simulink model "KalmanFilter(1)"  (R2024a)
settings: Solver=VariableStepAuto  StartTime=0.0  StopTime=1  RelTol=1e-3

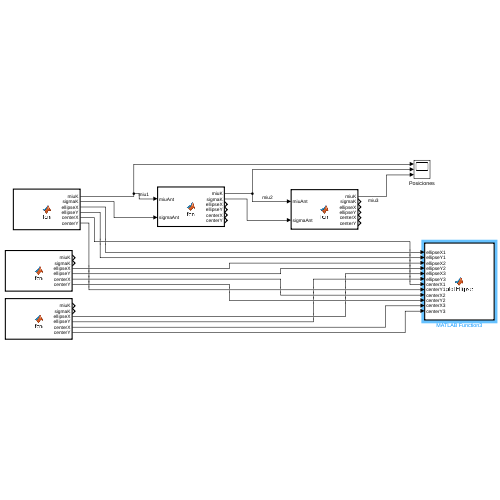
[thumbnail: Simulink's stored preview of the top-level diagram]
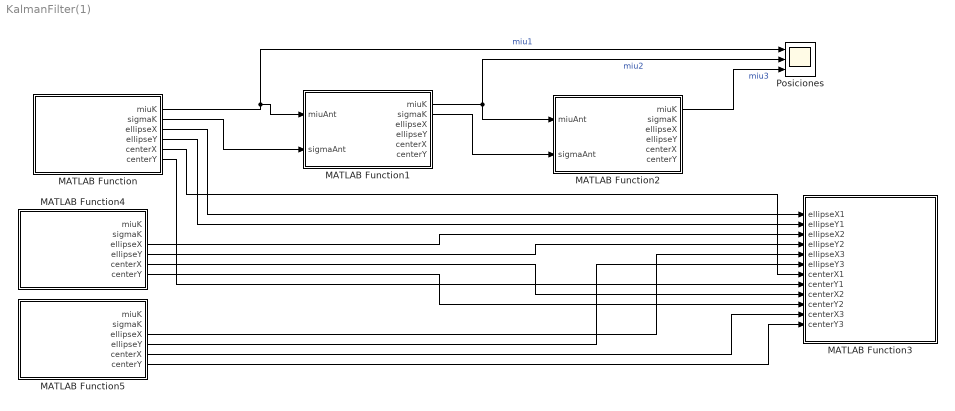
== system KalmanFilter(1) ==
  MATLAB Function : MATLAB Function  TreatAsAtomicUnit=on
  MATLAB Function1 : MATLAB Function  TreatAsAtomicUnit=on
  MATLAB Function2 : MATLAB Function  TreatAsAtomicUnit=on
  MATLAB Function3 : MATLAB Function  TreatAsAtomicUnit=on
  MATLAB Function4 : MATLAB Function  TreatAsAtomicUnit=on
  MATLAB Function5 : MATLAB Function  TreatAsAtomicUnit=on
  Posiciones : Scope  NumInputPorts=3
  wires:
  MATLAB Function/1(miuK) -> Posiciones/1, MATLAB Function1/1(miuAnt)  "miu1"
  MATLAB Function/2(sigmaK) -> MATLAB Function1/2(sigmaAnt)
  MATLAB Function1/1(miuK) -> Posiciones/2, MATLAB Function2/1(miuAnt)  "miu2"
  MATLAB Function1/2(sigmaK) -> MATLAB Function2/2(sigmaAnt)
  MATLAB Function2/1(miuK) -> Posiciones/3  "miu3"
  MATLAB Function/3(ellipseX) -> MATLAB Function3/1(ellipseX1)
  MATLAB Function/4(ellipseY) -> MATLAB Function3/2(ellipseY1)
  MATLAB Function/5(centerX) -> MATLAB Function3/7(centerX1)
  MATLAB Function/6(centerY) -> MATLAB Function3/8(centerY1)
  MATLAB Function4/3(ellipseX) -> MATLAB Function3/3(ellipseX2)
  MATLAB Function4/4(ellipseY) -> MATLAB Function3/4(ellipseY2)
  MATLAB Function4/5(centerX) -> MATLAB Function3/9(centerX2)
  MATLAB Function4/6(centerY) -> MATLAB Function3/10(centerY2)
  MATLAB Function5/3(ellipseX) -> MATLAB Function3/5(ellipseX3)
  MATLAB Function5/4(ellipseY) -> MATLAB Function3/6(ellipseY3)
  MATLAB Function5/5(centerX) -> MATLAB Function3/11(centerX3)
  MATLAB Function5/6(centerY) -> MATLAB Function3/12(centerY3)

== matlab function KalmanFilter(1)/MATLAB Function1 ==
  data: miuK output; sigmaK output; miuAnt input; sigmaAnt input; ellipseX output; ellipseY output; centerX output; centerY output
function [miuK, sigmaK, ellipseX, ellipseY, centerX, centerY]= fcn (miuAnt, sigmaAnt)

m = [3; 4]                      %Landmark position

QK = [0.5  0.01 0.01;           %Covariance Matrix - Motion(encoders)
      0.01 0.5  0.01;
      0.01 0.01 0.2]

RK = [0.1 0;                    %Covariance Matrix - Observation(LiDAR)
      0   0.02]
VK = 4 % m/s
WK = 4 % rad/s
deltaT = 0.1      %Time Sampling

z12 = [4.72; 0.72]
z13 = [4.69; 0.65]

%Step 2
miuK_est = [miuAnt(1) + deltaT * VK * cos(miuAnt(3));
            miuAnt(2) + deltaT * VK * sin(miuAnt(3));
            miuAnt(3) + deltaT * WK]
%Step 3
HK = [1 0 -deltaT * VK *sin(miuAnt(3));
      0 1 deltaT * VK *cos(miuAnt(3));
      0 0 1]

%Step 4 - Propagation of uncertainty
SigmaK = HK * sigmaAnt * HK' + QK

%Step 6 - Position Difference / Observation Model
deltaX = m(1) - miuK_est(1)
deltaY = m(2) - miuK_est(2)
p = (deltaX * deltaX) + (deltaY * deltaY)

ZK_est = [sqrt(p);                              
          atan2(deltaY, deltaX) - miuK_est(3)] 

%Step 7 - Linearise the observation model
GK = [-deltaX/sqrt(p) -deltaY/sqrt(p) 0;
      deltaY/p        -deltaX/p      -1]

%Step 8 - Second uncertainty Propagation
ZK = GK * SigmaK * GK' + RK

%Step 9 - Kalman Gain
Kk = SigmaK * GK' * inv(ZK)

%Step 10 - Position Calculation using real observation
miuK = miuK_est + Kk * (z12 -ZK_est)

%Step 11 - Get covariance
sigmaK = (eye(3) - Kk * GK) * QK

[ellipseX, ellipseY] = calculateEllipse(miuK(1:2), sigmaK(1:2, 1:2));
centerX = miuK(1);
centerY = miuK(2);
end

function [ellipseX, ellipseY] = calculateEllipse(mu, Sigma)
    theta = linspace(0, 2*pi, 100);
    [eig_vec, eig_val] = eig(Sigma);
    ellipse_points = [cos(theta); sin(theta)]' * sqrt(eig_val) * eig_vec';
    ellipseX = ellipse_points(:,1) + mu(1);
    ellipseY = ellipse_points(:,2) + mu(2);
end

== matlab function KalmanFilter(1)/MATLAB Function ==
  data: miuK output; sigmaK output; ellipseX output; ellipseY output; centerX output; centerY output
function [miuK, sigmaK, ellipseX, ellipseY, centerX, centerY]= fcn

%Miu = Position
miuAnt = [0; 0; 0]              %Robot First position
sigmaAnt = [0 0 0 ;             %Initial covariance matrix
            0 0 0; 
            0 0 0]              
m = [3; 4]                      %Landmark position

QK = [0.5  0.01 0.01;           %Covariance Matrix - Motion(encoders)
      0.01 0.5  0.01;
      0.01 0.01 0.2]

RK = [0.1 0;                    %Covariance Matrix - Observation(LiDAR)
      0   0.02]
VK = 1 % m/s
WK = 1 % rad/s
deltaT = 0.1      %Time Sampling

z11 = [4.87; 0.8]
z12 = [4.72; 0.72]
z13 = [4.69; 0.65]

%Step 2
miuK_est = [miuAnt(1) + deltaT * VK * cos(miuAnt(3));
            miuAnt(2) + deltaT * VK * sin(miuAnt(3));
            miuAnt(3) + deltaT * WK]
%Step 3
HK = [1 0 -deltaT * VK *sin(miuAnt(3));
      0 1 deltaT * VK *cos(miuAnt(3));
      0 0 1]

%Step 4 - Propagation of uncertainty
SigmaK = HK * sigmaAnt * HK' + QK

%Step 6 - Position Difference / Observation Model
deltaX = m(1) - miuK_est(1)
deltaY = m(2) - miuK_est(2)
p = (deltaX * deltaX) + (deltaY * deltaY)

ZK_est = [sqrt(p);                              
          atan2(deltaY, deltaX) - miuK_est(3)] 

%Step 7 - Linearise the observation model
GK = [-deltaX/sqrt(p) -deltaY/sqrt(p) 0;
      deltaY/p        -deltaX/p      -1]

%Step 8 - Second uncertainty Propagation
ZK = GK * SigmaK * GK' + RK

%Step 9 - Kalman Gain
Kk = SigmaK * GK' * inv(ZK)
%Step 10 - Position Calculation using real observation
miuK = miuK_est + Kk * (z11 -ZK_est)

%Step 11 - Get covariance
sigmaK = (eye(3) - Kk * GK) * QK

[ellipseX, ellipseY] = calculateEllipse(miuK(1:2), sigmaK(1:2, 1:2));
centerX = miuK(1);
centerY = miuK(2);
end

function [ellipseX, ellipseY] = calculateEllipse(mu, Sigma)
    theta = linspace(0, 2*pi, 100);
    [eig_vec, eig_val] = eig(Sigma);
    ellipse_points = [cos(theta); sin(theta)]' * sqrt(eig_val) * eig_vec';
    ellipseX = ellipse_points(:,1) + mu(1);
    ellipseY = ellipse_points(:,2) + mu(2);
end

== matlab function KalmanFilter(1)/MATLAB Function2 ==
  data: miuK output; sigmaK output; miuAnt input; sigmaAnt input; ellipseX output; ellipseY output; centerX output; centerY output
function [miuK, sigmaK, ellipseX, ellipseY, centerX, centerY]= fcn (miuAnt, sigmaAnt)

m = [3; 4]                      %Landmark position

QK = [0.5  0.01 0.01;           %Covariance Matrix - Motion(encoders)
      0.01 0.5  0.01;
      0.01 0.01 0.2]

RK = [0.1 0;                    %Covariance Matrix - Observation(LiDAR)
      0   0.02]
VK = 4 % m/s
WK = 4 % rad/s
deltaT = 0.1      %Time Sampling

z13 = [4.69; 0.65]

%Step 2
miuK_est = [miuAnt(1) + deltaT * VK * cos(miuAnt(3));
            miuAnt(2) + deltaT * VK * sin(miuAnt(3));
            miuAnt(3) + deltaT * WK]
%Step 3
HK = [1 0 -deltaT * VK *sin(miuAnt(3));
      0 1 deltaT * VK *cos(miuAnt(3));
      0 0 1]

%Step 4 - Propagation of uncertainty
SigmaK = HK * sigmaAnt * HK' + QK

%Step 6 - Position Difference / Observation Model
deltaX = m(1) - miuK_est(1)
deltaY = m(2) - miuK_est(2)
p = (deltaX * deltaX) + (deltaY * deltaY)

ZK_est = [sqrt(p);                              
          atan2(deltaY, deltaX) - miuK_est(3)] 

%Step 7 - Linearise the observation model
GK = [-deltaX/sqrt(p) -deltaY/sqrt(p) 0;
      deltaY/p        -deltaX/p      -1]

%Step 8 - Second uncertainty Propagation
ZK = GK * SigmaK * GK' + RK

%Step 9 - Kalman Gain
Kk = SigmaK * GK' * inv(ZK)

%Step 10 - Position Calculation using real observation
miuK = miuK_est + Kk * (z13 -ZK_est)

%Step 11 - Get covariance
sigmaK = (eye(3) - Kk * GK) * QK

[ellipseX, ellipseY] = calculateEllipse(miuK(1:2), sigmaK(1:2, 1:2));
centerX = miuK(1);
centerY = miuK(2);
end

function [ellipseX, ellipseY] = calculateEllipse(mu, Sigma)
    theta = linspace(0, 2*pi, 100);
    [eig_vec, eig_val] = eig(Sigma);
    ellipse_points = [cos(theta); sin(theta)]' * sqrt(eig_val) * eig_vec';
    ellipseX = ellipse_points(:,1) + mu(1);
    ellipseY = ellipse_points(:,2) + mu(2);
end

== matlab function KalmanFilter(1)/MATLAB Function3 ==
  data: ellipseX1 input; ellipseY1 input; ellipseX2 input; ellipseY2 input; ellipseX3 input; ellipseY3 input; centerX1 input; centerY1 input; centerX2 input; centerY2 input; centerX3 input; centerY3 input
function plotEllipse(ellipseX1, ellipseY1, ellipseX2, ellipseY2, ellipseX3, ellipseY3, centerX1, centerY1, centerX2, centerY2, centerX3, centerY3)
    % Check if the figure is already open
    existing_figures = findall(0, 'Type', 'figure');
    if isempty(existing_figures)
        figure;
    else
        figure(existing_figures(1)); % Use the first existing figure
    end
    
    hold on;
    
    % Plot the first ellipse
    plot(ellipseX1, ellipseY1, 'b-');
    plot(centerX1, centerY1, 'bo', 'MarkerSize', 10, 'LineWidth', 2); % Centro de la elipse 1
    
    % Plot the second ellipse
    plot(ellipseX2, ellipseY2, 'r-');
    plot(centerX2, centerY2, 'ro', 'MarkerSize', 10, 'LineWidth', 2); % Centro de la elipse 2
    
    % Plot the third ellipse
    plot(ellipseX3, ellipseY3, 'g-');
    plot(centerX3, centerY3, 'go', 'MarkerSize', 10, 'LineWidth', 2); % Centro de la elipse 3
    
    hold off;
    xlabel('X');
    ylabel('Y');
    title('Confidence Ellipses');
    axis equal;
    grid on;
    legend('Ellipse 1 - Original', 'Center 1', 'Ellipse 2 - Qk Double Values', 'Center 2', 'Ellipse 3 - Rk double values', 'Center 3');
end

== matlab function KalmanFilter(1)/MATLAB Function4 ==
  data: miuK output; sigmaK output; ellipseX output; ellipseY output; centerX output; centerY output
function [miuK, sigmaK, ellipseX, ellipseY, centerX, centerY]= fcn

%Miu = Position
miuAnt = [0; 0; 0]              %Robot First position
sigmaAnt = [0 0 0 ;             %Initial covariance matrix
            0 0 0; 
            0 0 0]              
m = [3; 4]                      %Landmark position

QK = [1.0  0.01 0.01;           %Covariance Matrix - Motion(encoders)
      0.01 1.0  0.01;
      0.01 0.01 0.4]

RK = [0.1 0;                    %Covariance Matrix - Observation(LiDAR)
      0   0.02]
VK = 1 % m/s
WK = 1 % rad/s
deltaT = 0.1      %Time Sampling

z11 = [4.87; 0.8]
z12 = [4.72; 0.72]
z13 = [4.69; 0.65]

%Step 2
miuK_est = [miuAnt(1) + deltaT * VK * cos(miuAnt(3));
            miuAnt(2) + deltaT * VK * sin(miuAnt(3));
            miuAnt(3) + deltaT * WK]
%Step 3
HK = [1 0 -deltaT * VK *sin(miuAnt(3));
      0 1 deltaT * VK *cos(miuAnt(3));
      0 0 1]

%Step 4 - Propagation of uncertainty
SigmaK = HK * sigmaAnt * HK' + QK

%Step 6 - Position Difference / Observation Model
deltaX = m(1) - miuK_est(1)
deltaY = m(2) - miuK_est(2)
p = (deltaX * deltaX) + (deltaY * deltaY)

ZK_est = [sqrt(p);                              
          atan2(deltaY, deltaX) - miuK_est(3)] 

%Step 7 - Linearise the observation model
GK = [-deltaX/sqrt(p) -deltaY/sqrt(p) 0;
      deltaY/p        -deltaX/p      -1]

%Step 8 - Second uncertainty Propagation
ZK = GK * SigmaK * GK' + RK

%Step 9 - Kalman Gain
Kk = SigmaK * GK' * inv(ZK)
%Step 10 - Position Calculation using real observation
miuK = miuK_est + Kk * (z11 -ZK_est)

%Step 11 - Get covariance
sigmaK = (eye(3) - Kk * GK) * QK

[ellipseX, ellipseY] = calculateEllipse(miuK(1:2), sigmaK(1:2, 1:2));
centerX = miuK(1);
centerY = miuK(2);
end

function [ellipseX, ellipseY] = calculateEllipse(mu, Sigma)
    theta = linspace(0, 2*pi, 100);
    [eig_vec, eig_val] = eig(Sigma);
    ellipse_points = [cos(theta); sin(theta)]' * sqrt(eig_val) * eig_vec';
    ellipseX = ellipse_points(:,1) + mu(1);
    ellipseY = ellipse_points(:,2) + mu(2);
end

== matlab function KalmanFilter(1)/MATLAB Function5 ==
  data: miuK output; sigmaK output; ellipseX output; ellipseY output; centerX output; centerY output
function [miuK, sigmaK, ellipseX, ellipseY, centerX, centerY]= fcn

%Miu = Position
miuAnt = [0; 0; 0]              %Robot First position
sigmaAnt = [0 0 0 ;             %Initial covariance matrix
            0 0 0; 
            0 0 0]              
m = [3; 4]                      %Landmark position

QK = [0.5  0.01 0.01;           %Covariance Matrix - Motion(encoders)
      0.01 0.5  0.01;
      0.01 0.01 0.2]

RK = [0.2 0;                    %Covariance Matrix - Observation(LiDAR)
      0   0.04]
VK = 1 % m/s
WK = 1 % rad/s
deltaT = 0.1      %Time Sampling

z11 = [4.87; 0.8]
z12 = [4.72; 0.72]
z13 = [4.69; 0.65]

%Step 2
miuK_est = [miuAnt(1) + deltaT * VK * cos(miuAnt(3));
            miuAnt(2) + deltaT * VK * sin(miuAnt(3));
            miuAnt(3) + deltaT * WK]
%Step 3
HK = [1 0 -deltaT * VK *sin(miuAnt(3));
      0 1 deltaT * VK *cos(miuAnt(3));
      0 0 1]

%Step 4 - Propagation of uncertainty
SigmaK = HK * sigmaAnt * HK' + QK

%Step 6 - Position Difference / Observation Model
deltaX = m(1) - miuK_est(1)
deltaY = m(2) - miuK_est(2)
p = (deltaX * deltaX) + (deltaY * deltaY)

ZK_est = [sqrt(p);                              
          atan2(deltaY, deltaX) - miuK_est(3)] 

%Step 7 - Linearise the observation model
GK = [-deltaX/sqrt(p) -deltaY/sqrt(p) 0;
      deltaY/p        -deltaX/p      -1]

%Step 8 - Second uncertainty Propagation
ZK = GK * SigmaK * GK' + RK

%Step 9 - Kalman Gain
Kk = SigmaK * GK' * inv(ZK)
%Step 10 - Position Calculation using real observation
miuK = miuK_est + Kk * (z11 -ZK_est)

%Step 11 - Get covariance
sigmaK = (eye(3) - Kk * GK) * QK

[ellipseX, ellipseY] = calculateEllipse(miuK(1:2), sigmaK(1:2, 1:2));
centerX = miuK(1);
centerY = miuK(2);
end

function [ellipseX, ellipseY] = calculateEllipse(mu, Sigma)
    theta = linspace(0, 2*pi, 100);
    [eig_vec, eig_val] = eig(Sigma);
    ellipse_points = [cos(theta); sin(theta)]' * sqrt(eig_val) * eig_vec';
    ellipseX = ellipse_points(:,1) + mu(1);
    ellipseY = ellipse_points(:,2) + mu(2);
end
